simulink model "eepromBuffer"  (R2018a)
settings: Solver=FixedStepAuto  StartTime=0.0  StopTime=100  FixedStep=0.0001  RelTol=1e-3
settings Model: EnablePacing=on  PacingRate=0.180000  Creator=SIMONE  LastModifiedBy=SIMONE
settings SFSimCC: SimCustomHeaderCode="#include \"id_can.h\""

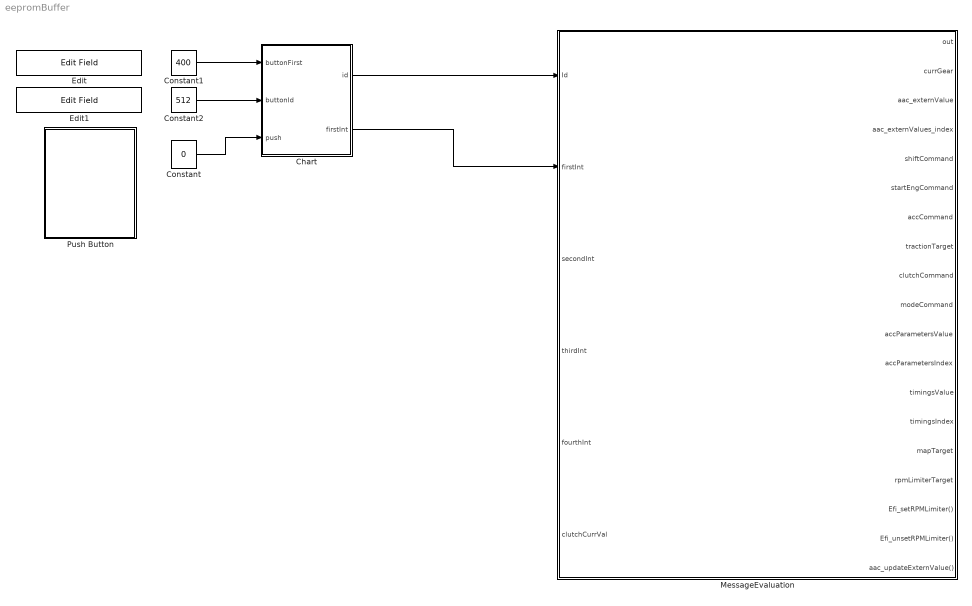
== system eepromBuffer ==
  Chart : Stateflow chart  TreatAsAtomicUnit=on
  Constant : Constant  Value=0  VectorParams1D=off
  Constant1 : Constant  Value=400  OutDataTypeStr=uint16
  Constant2 : Constant  Value=512  OutDataTypeStr=uint16
  Edit : EditField  WebBlockId=65  LabelPosition=Hide  Alignment=Center
  Edit1 : EditField  WebBlockId=66  LabelPosition=Hide  Alignment=Center
  MessageEvaluation : Stateflow chart  TreatAsAtomicUnit=on  SystemSampleTime=[0.001, 0.0002]
  Push Button : Subsystem  DialogController=hmiCreateDDGDialog  IsWebBlock=on  mask(MWDashboardBlock){webBlockId=e6adbf7e-c019-4fe3-b011-d8f1e3f1f276, webBlockType=pushbutton, ShowInLibBrwoser=on, ShowInitialText=on, HMISrcModelName=GCU_CAN_C}
      mask prompts: webBlockId "WebBlock Id"; webBlockType "WebBlock Type"; HMISrcModelName "Source Model"
      mask help: SimulinkHMI:dialogs:PushButtonDialogDesc
      mask Help: helpview([docroot '/mapfiles/simulink.map'], 'hmi_push_button')
      mask Display:
      | model = bdroot(gcb);
      | if strcmp(get_param(model,'BlockDiagramType'), 'library')
      |     image([(matlabroot) '/toolbox/simulink/hmi/icons/PushButton.png']);
      | end
  wires:
  Chart/1(id) -> MessageEvaluation/1(Id)
  Constant/1 -> Chart/3(push)
  Constant1/1 -> Chart/1(buttonFirst)
  Constant2/1 -> Chart/2(buttonId)
  Chart/2(firstInt) -> MessageEvaluation/2(firstInt)

== system eepromBuffer/Push Button ==

== stateflow chart eepromBuffer/Chart ==
  state b
    entry:
    id=buttonId;
    firstInt = buttonFirst;
    during:
    id=0;
    firstInt=0;
  state a
    entry:
    id=0;
    firstInt=0;
  (default) -> a
  a -> b : [push==1]
  b -> a : [push==0]
  data: id output uint16 size=1 =uint16(500); buttonFirst input uint16; buttonId input uint16; push input; firstInt output uint16

== stateflow chart eepromBuffer/MessageEvaluation ==
  state sendStartEngCommand [function]
    (default) -> (junction 280)
    (junction 280) -> (junction 281) [order 1] : [startEngCommand >= 255]
    (junction 280) -> (junction 282) [order 2] : {startEngCommand = startEngCommand + 1;}
    (junction 281) -> (junction 283) : {startEngCommand = 0}
  state GEAR_RPM_UPDATE [group]
    (junction 498) -> (junction 499) : { currGear = firstInt;
        |   aac_externValues_index = uint16(aac_values.RPM);
        |   aac_externValue = secondInt;
        |   send(aac_updateExternValue);}
  state START_ENGINE [group]
    (junction 502) -> (junction 503) : {sendStartEngCommand();}
  state sendShiftCommand(com) [function]
    note: QUESTO CONTROLLO VOGLIO SPOSTARLO IN TIMER
    (default) -> (junction 211)
    (junction 211) -> (junction 212) [order 1] : [shiftCommand[0] >= 255]
    (junction 211) -> (junction 214) [order 2] : {shiftCommand[0] = shiftCommand[0] + 1}
    (junction 212) -> (junction 215) : {shiftCommand[0] = 0}
    (junction 214) -> (junction 215)
    (junction 215) -> (junction 216) : {shiftCommand[1] = com}
    (junction 216) -> (junction 224) [order 1] : [clutchCurrVal ~= 100]
    (junction 216) -> (junction 229) [order 2]
    (junction 224) -> (junction 226)
    (junction 226) -> (junction 305) [order 1] : [(com == GEAR_COMMAND_NEUTRAL_UP) || (com == GEAR_COMMAND_NEUTRAL_DOWN) ||  (com == GEAR_COMMAND_DOWN) ]
    (junction 305) -> (junction 309) : {sendAccCommand(STOP_COM)}
    (junction 226) -> (junction 307) [order 2]
  state SW_GEARSHIFT [group]
    (junction 504) -> (junction 506) : {sendShiftCommand(firstInt);}
  note: id non è più valido
  state WHEEL_SPEED_UPDATE [group]
    (junction 508) -> (junction 541) : { aac_externValues_index = uint16(aac_values.WHEEL_SPEED)
        |   aac_externValue = firstInt/10;
        |   send(aac_updateExternValue);}
  state sendClutchCommand(com) [function]
    (default) -> (junction 187)
    (junction 187) -> (junction 188) [order 1] : [clutchCommand[0] >= 255]
    (junction 187) -> (junction 190) [order 2] : {clutchCommand[0] = clutchCommand[0] + 1}
    (junction 188) -> (junction 191) : {clutchCommand[0] = 0}
    (junction 190) -> (junction 191)
    (junction 191) -> (junction 192) : {clutchCommand[1] = com}
  state SET_CLUTCH_MODE_MAP [group]
    (junction 511) -> (junction 512) : {clutchTarget = firstInt;
        |  sendModeCommand(secondInt);
        |  mapTarget = thirdInt;}
    (junction 512) -> (junction 552) [order 1] : [clutchTarget > ACC_CLUTCH_NOISE_LEVEL]
    (junction 512) -> (junction 553) [order 2]
    (junction 552) -> (junction 544) : {sendAccCommand(STOP_COM);}
    (junction 553) -> (junction 544)
    (junction 544) -> (junction 548) : {sendClutchCommand(clutchTarget);}
  state sendAccCommand(com) [function]
    (default) -> (junction 164)
    (junction 164) -> (junction 167) [order 1] : [accCommand[0] >= 255]
    (junction 164) -> (junction 171) [order 2] : {accCommand[0] = accCommand[0] + 1}
    (junction 167) -> (junction 169) : {accCommand[0] = 0}
    (junction 169) -> (junction 173)
    (junction 171) -> (junction 173)
    (junction 173) -> (junction 176) : {accCommand[1] = com}
  state ACC_COM [group]
    (junction 560) -> (junction 558) : {sendAccCommand(firstInt);}
    (junction 558) -> (junction 562) [order 1] : [accCommand[1] == STOP_COM]
    (junction 558) -> (junction 564) [order 2]
    (junction 562) -> (junction 561) : {sendClutchCommand(uint8(0))}
  state sendModeCommand(com) [function]
    (default) -> (junction 324)
    (junction 324) -> (junction 325) [order 1] : [modeCommand[0] >= 255]
    (junction 324) -> (junction 327) [order 2] : {modeCommand[0] = modeCommand[0] + 1}
    (junction 325) -> (junction 328) : {modeCommand[0] = 0}
    (junction 327) -> (junction 328)
    (junction 328) -> (junction 329) : {modeCommand[1] = com}
  state SET_TRACTION_RPM_LIMITER [group]
    (junction 518) -> (junction 519) : {tractionTarget = uint16(firstInt) * 100;
        |  rpmLimiterTarget;}
  state SET_AUTOGEARSHIFT [group]
    (junction 588) -> (junction 589)
  state READ_EEPROM [group] [commented out]
    (junction 527) -> (junction 528) [commented out]
  state WRITE_EEPROM [group] [commented out]
    (junction 530) -> (junction 531) [commented out] : {accParametersIndex = firstInt;
        |  accParametersValue = secondInt;
        |  timingsIndex = thirdInt;
        |  timingsValue = fourthInt;}
  (default) -> (junction 389)
  (junction 389) -> (junction 498) [order 1] : [Id == EFI_GEAR_RPM_TPS_PH2O_ID]
  (junction 389) -> (junction 423) [order 2]
  (junction 423) -> (junction 502) [order 1] : [Id == SW_FIRE_GCU_ID]
  (junction 423) -> (junction 405) [order 2]
  (junction 405) -> (junction 504) [order 1] : [Id == SW_GEARSHIFT_ID]
  (junction 405) -> (junction 383) [order 2]
  (junction 383) -> (junction 508) [order 1] : [Id == EFI_TRACTION_CONTROL_ID]
  (junction 383) -> (junction 390) [order 2]
  (junction 390) -> (junction 511) [order 1] : [Id==SW_CLUTCH_MODE_MAP_GCU_ID]
  (junction 390) -> (junction 426) [order 2]
  (junction 426) -> (junction 560) [order 1] : [Id == SW_OK_BUTTON_GCU_ID]
  (junction 426) -> (junction 398) [order 2]
  (junction 398) -> (junction 518) [order 1] : [Id == SW_TRACTION_LIMITER_GCU_ID]
  (junction 398) -> (junction 586) [order 2]
  (junction 586) -> (junction 588) [order 1] : [Id==DCU_AUTOGEARSHIFT_GCU_ID]
  (junction 586) -> (junction 593) [order 2]
  (junction 428) -> (junction 527) [commented out] : [Id == EEPROM_READ_ID]
  (junction 428) -> (junction 379) [commented out]
  (junction 379) -> (junction 530) [commented out] : [Id == EEPROM_WRITE_ID]
  (junction 379) -> (junction 574) [commented out]
  data: STOP_COM constant uint16 =uint16(0); com function_input uint16 size=1; STOP_COM constant uint16 =uint16(0); GEAR_COMMAND_NEUTRAL_DOWN constant uint16 =uint16(100); GEAR_COMMAND_NEUTRAL_UP constant uint16 =uint16(50); GEAR_COMMAND_DOWN constant uint16 =uint16(200); com function_input uint16 size=1; clutchTarget local uint8 size=1; STOP_COM constant uint16 =uint16(0); ACC_CLUTCH_NOISE_LEVEL constant uint8 =uint8(30); com function_input uint16 size=1; STOP_COM constant uint16 =uint16(0); STOP_COM constant uint16 =uint16(0); com function_input uint16 size=1; Id input uint16 size=1; firstInt input uint16 size=1; secondInt input uint16 size=1; thirdInt input uint16 size=1; fourthInt input uint16 size=1; out output size=1 =0; currGear output uint16 size=1 [..uint16(5)] =uint16(0); aac_externValue output uint16 size=1 =uint16(0); aac_externValues_index output uint16 size=1 [..uint16(3)] =uint16(0); shiftCommand output uint16 size=[1, 2] =[uint16(0), uint16(0)]; startEngCommand output uint8 size=1 =uint8(0); accCommand output uint16 size=[1,2] =[uint16(0), uint16(0)]; tractionTarget output uint16 size=1; clutchCommand output uint8 size=[1,2] =[uint8(0), uint8(0)]; clutchCurrVal input uint8 size=1; modeCommand output uint16 size=[1,2] =[uint16(0), uint16(0)]; accParametersValue output uint16 size=1 =uint16(0); accParametersIndex output uint16 size=1 [..uint16(3)] =uint16(0); timingsValue output uint16 size=1 =uint16(0); timingsIndex output uint16 size=1 [..uint16(3)] =uint16(0); mapTarget output uint16 size=1 [..uint16(5)] =uint16(0); rpmLimiterTarget output uint16 size=1
  events: Efi_setRPMLimiter output FUNCTION_CALL_EVENT; Efi_unsetRPMLimiter output FUNCTION_CALL_EVENT; aac_updateExternValue output FUNCTION_CALL_EVENT
